simulink library "csc_emp_est_mass_props_lib"  (R2015b)
settings: Solver=ode45  StartTime=0.0  StopTime=10.0  RelTol=1e-3
values from neighbouring files (symbols this model uses):
  emp_initial_fuel_used = 0    [csc_emp_est_mass_props_init.m]
  emp_mass_fillfrac_0 = 30.0    (= 30)    [csc_emp_est_mass_props_init.m]
  emp_max_fuel_used = emp_mass_fillfrac_100 - emp_mass_fillfrac_0    (= 542.9)    [csc_emp_est_mass_props_init.m]
  emp_min_fuel_used = 0    [csc_emp_est_mass_props_init.m]
  emp_rp1_to_htp_ratio = 1/7.5    (= 0.133333333333)    [csc_emp_est_mass_props_init.m]
undefined symbols (not defined in the file or in its folder): DiscIntNeverNeededParam, emp_biprop_gISP_inverse, emp_cg_wet_dry_x, emp_cg_wet_dry_y, emp_cg_wet_dry_z, emp_coarse_gISP_inverse, emp_fine_gISP_inverse, emp_mass_wet_dry, emp_mono_gISP_inverse, emp_time_to_biprop_thrust, emp_time_to_coarse_thrust, emp_time_to_fine_thrust, emp_time_to_mono_thrust
libraries: simulink x3, util_info_lib x1, util_common_lib x1
settings Model: Creator=escrane  LastModifiedBy=jimkaidy
settings DataIOCC: SaveFormat=Array
settings DebuggingCC: UnderspecifiedInitializationDetection=Classic  MergeDetectMultiDrivingBlocksExec=none  SolverPrmCheckMsg=warning  StateNameClashWarn=warning
settings HardwareCC: ProdBitPerPointer=32  ProdLargestAtomicFloat=None  ProdIntDivRoundTo=Undefined  ProdEndianess=Unspecified  ProdWordSize=32  ProdHWDeviceType=32-bit Generic
settings GRTTargetCC: GeneratePreprocessorConditionals=Disable all
settings ConfigComp: CovModelRefEnable=Off  CovSFcnEnable=off

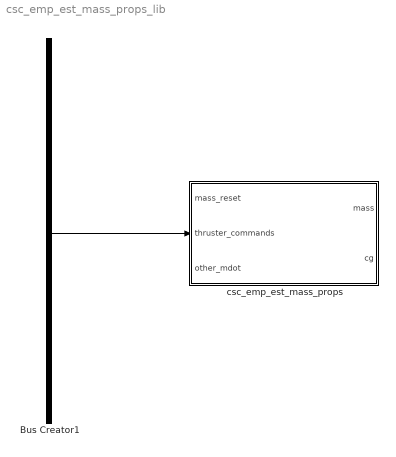
== system csc_emp_est_mass_props_lib ==
  Bus Creator1 : BusCreator  Inputs=26  OutDataTypeStr=Bus: cnt_lander_bus_msg  NonVirtualBus=on
  csc_emp_est_mass_props : Subsystem
  wires:
  ? -> Bus Creator1/1  "cnt_thruster1_time"
  ? -> Bus Creator1/3  "cnt_thruster3_time"
  ? -> Bus Creator1/2  "cnt_thruster2_time"
  ? -> Bus Creator1/5  "cnt_thruster5_time"
  ? -> Bus Creator1/4  "cnt_thruster4_time"
  ? -> Bus Creator1/6  "cnt_thruster6_time"
  ? -> Bus Creator1/13  "cnt_thruster13_time"
  ? -> Bus Creator1/16  "cnt_thruster16_time"
  ? -> Bus Creator1/20  "cnt_thruster20_time"
  ? -> Bus Creator1/17  "cnt_thruster17_time"
  ? -> Bus Creator1/8  "cnt_thruster8_time"
  ? -> Bus Creator1/9  "cnt_thruster9_time"
  ? -> Bus Creator1/10  "cnt_thruster10_time"
  ? -> Bus Creator1/7  "cnt_thruster7_time"
  ? -> Bus Creator1/11  "cnt_thruster11_time"
  ? -> Bus Creator1/23  "cnt_thruster23_time"
  ? -> Bus Creator1/14  "cnt_thruster14_time"
  ? -> Bus Creator1/12  "cnt_thruster12_time"
  ? -> Bus Creator1/19  "cnt_thruster19_time"
  ? -> Bus Creator1/24  "cnt_thruster24_time"
  ? -> Bus Creator1/15  "cnt_thruster15_time"
  ? -> Bus Creator1/21  "cnt_thruster21_time"
  ? -> Bus Creator1/22  "cnt_thruster22_time"
  ? -> Bus Creator1/18  "cnt_thruster18_time"
  ? -> Bus Creator1/26  "main_biprop_monoprop"
  Bus Creator1/1 -> csc_emp_est_mass_props/2(thruster_commands)
  ? -> Bus Creator1/25  "main_thruster_cmd"

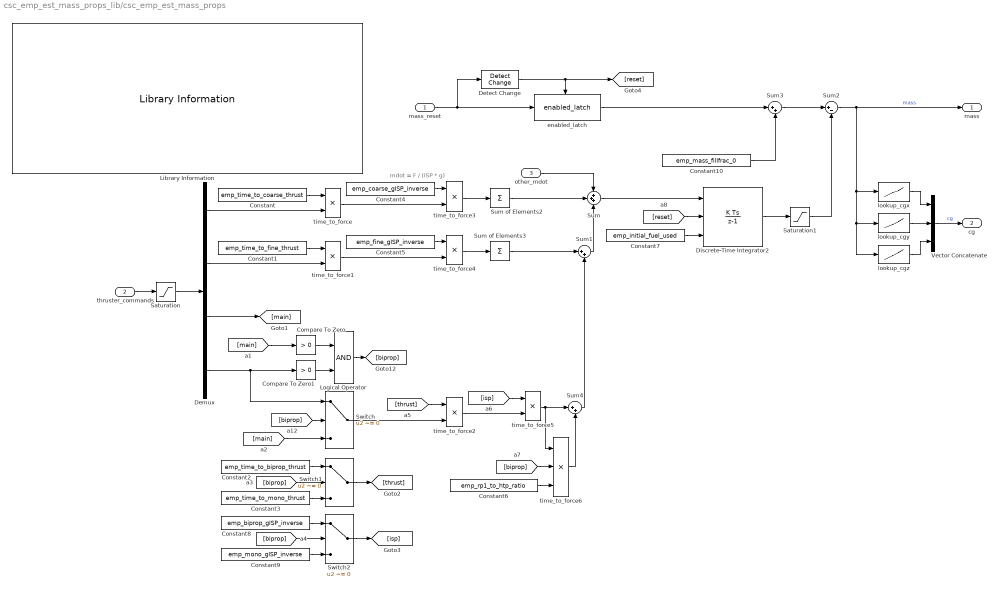
== system csc_emp_est_mass_props_lib/csc_emp_est_mass_props ==
  note: mdot = F / (ISP * g)
  mass_reset : Inport
  thruster_commands : Inport  Port=2
  "other_mdot " : Inport  Port=3
  Compare To Zero : simulink/Logic and Bit Operations/Compare To Zero  relop=>  OutDataTypeStr=boolean
  Compare To Zero1 : simulink/Logic and Bit Operations/Compare To Zero  relop=>  OutDataTypeStr=boolean
  Constant : Constant  Value=emp_time_to_coarse_thrust
  Constant1 : Constant  Value=emp_time_to_fine_thrust
  Constant10 : Constant  Value=emp_mass_fillfrac_0
  Constant2 : Constant  Value=emp_time_to_biprop_thrust
  Constant3 : Constant  Value=emp_time_to_mono_thrust
  Constant4 : Constant  Value=emp_coarse_gISP_inverse
  Constant5 : Constant  Value=emp_fine_gISP_inverse
  Constant6 : Constant  Value=emp_rp1_to_htp_ratio
  Constant7 : Constant  Value=emp_initial_fuel_used
  Constant8 : Constant  Value=emp_biprop_gISP_inverse
  Constant9 : Constant  Value=emp_mono_gISP_inverse
  Demux : Demux  Outputs=[12 12 1 1]
  Detect Change : simulink/Logic and Bit Operations/Detect Change  vinit=0  InputProcessing=Inherited  OutDataTypeStr=boolean
  Discrete-Time Integrator2 : DiscreteIntegrator  gainval=1  ExternalReset=rising  InitialConditionSource=external  SampleTime=-1  ICPrevOutput=DiscIntNeverNeededParam  ICPrevScaledInput=DiscIntNeverNeededParam
  Library Information : util_info_lib/Library Information  owner='escrane'
  Logical Operator : Logic  AllPortsSameDT=off  OutDataTypeStr=boolean
  Saturation : Saturate  UpperLimit=100  LowerLimit=0
  Saturation1 : Saturate  UpperLimit=emp_max_fuel_used  LowerLimit=emp_min_fuel_used
  Sum : Sum  Inputs=+++
  Sum of Elements2 : Sum  Inputs=+
  Sum of Elements3 : Sum  Inputs=+
  Sum1 : Sum  Inputs=|++
  Sum2 : Sum  Inputs=|+-
  Sum3 : Sum  Inputs=|++
  Sum4 : Sum  Inputs=|++
  Switch : Switch  Criteria=u2 ~= 0
  Switch1 : Switch  Criteria=u2 ~= 0
  Switch2 : Switch  Criteria=u2 ~= 0
  Vector Concatenate : Concatenate  NumInputs=3
  enabled_latch : util_common_lib/enabled_latch  initial_output=emp_initial_fuel_load
  lookup_cgx : Lookup  InputValues=emp_mass_wet_dry  Table=emp_cg_wet_dry_x
  lookup_cgy : Lookup  InputValues=emp_mass_wet_dry  Table=emp_cg_wet_dry_y
  lookup_cgz : Lookup  InputValues=emp_mass_wet_dry  Table=emp_cg_wet_dry_z
  time_to_force{,1..5} (6 alike) : Product  RndMeth=Zero
  time_to_force6 : Product  Inputs=3  RndMeth=Zero
  mass : Outport
  cg : Outport  Port=2
  wires:
  enabled_latch/1 -> Sum3/1
  Detect Change/1 -> [reset], enabled_latch/Enable
  Constant10/1 -> Sum3/2
  mass_reset/1 -> enabled_latch/1, Detect Change/1
  "other_mdot "/1 -> Sum/1
  Sum4/1 -> Sum1/2
  Saturation/1 -> Demux/1
  Constant/1 -> time_to_force/1
  thruster_commands/1 -> Saturation/1
  [biprop] -> Switch/2
  Logical Operator/1 -> [biprop]
  Compare To Zero/1 -> Logical Operator/1
  Compare To Zero1/1 -> Logical Operator/2
  Demux/4 -> Switch/1, Compare To Zero1/1
  Demux/3 -> [main]
  [main] -> Compare To Zero/1
  [main] -> Switch/3
  Demux/1 -> time_to_force/2
  Constant1/1 -> time_to_force1/1
  Demux/2 -> time_to_force1/2
  [biprop] -> Switch1/2
  Constant2/1 -> Switch1/1
  Constant3/1 -> Switch1/3
  time_to_force/1 -> time_to_force3/2
  Constant4/1 -> time_to_force3/1
  time_to_force3/1 -> Sum of Elements2/1
  time_to_force1/1 -> time_to_force4/2
  Constant5/1 -> time_to_force4/1
  time_to_force4/1 -> Sum of Elements3/1
  Sum of Elements2/1 -> Sum/2
  time_to_force2/1 -> time_to_force5/2
  [isp] -> time_to_force5/1
  [biprop] -> Switch2/2
  Constant8/1 -> Switch2/1
  Constant9/1 -> Switch2/3
  Switch1/1 -> [thrust]
  Switch2/1 -> [isp]
  Switch/1 -> time_to_force2/2
  [thrust] -> time_to_force2/1
  Sum of Elements3/1 -> Sum1/1
  Sum1/1 -> Sum/3
  Sum/1 -> Discrete-Time Integrator2/1
  [reset] -> Discrete-Time Integrator2/2
  Constant7/1 -> Discrete-Time Integrator2/3
  Sum3/1 -> Sum2/1
  Discrete-Time Integrator2/1 -> Saturation1/1
  Sum2/1 -> lookup_cgy/1, lookup_cgz/1, lookup_cgx/1, mass/1  "mass"
  Vector Concatenate/1 -> cg/1  "cg"
  lookup_cgz/1 -> Vector Concatenate/3
  lookup_cgy/1 -> Vector Concatenate/2
  lookup_cgx/1 -> Vector Concatenate/1
  Saturation1/1 -> Sum2/2
  Constant6/1 -> time_to_force6/3
  [biprop] -> time_to_force6/2
  time_to_force5/1 -> Sum4/1, time_to_force6/1
  time_to_force6/1 -> Sum4/2
